simulink model "model6"  (R2022a)
settings: Solver=VariableStepAuto  StartTime=0.0  StopTime=10.0  RelTol=1e-3
values from neighbouring files (symbols this model uses):
  A = [0 0 0 1 0 0; 0 0 0 0 1 0; 0 0 0 0 0 1; 0 6.5 -10 -alpha 0 0; a_51 a_52 a_53 a_54 a_55 a_56; 5 -3.6 0 0 0 -gamma]    [ME5401.m]
  B = [0 0; 0 0; 0 0; beta 11.2; b_51 b_52; 40 delta]    [ME5401.m]    (also in unity_place.m = B*q)
  C = [1 0 0 0 0 0; 0 1 0 0 0 0; 0 0 1 0 0 0]    [ME5401.m]    (also in place_pole.m = CC; unity_place.m = W_c)
  K_2 = my_lqr(A,B,Q,R)    [ME5401.m]
settings Model: Creator=jiaya  LastModifiedBy=jiaya
settings ModelReferenceCC: EnableRefExpFcnMdlSchedulingChecks=off
settings RTWCC: Description=Generic Real-Time Target

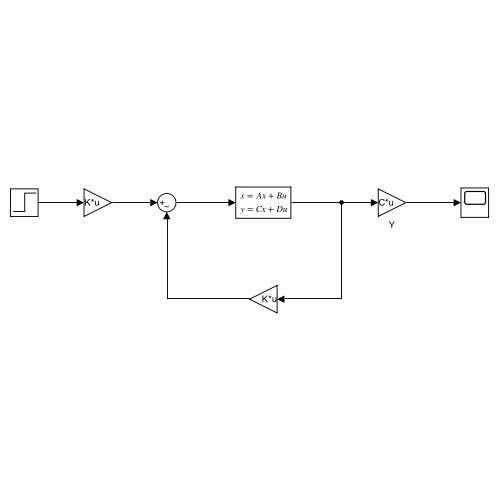
[thumbnail: Simulink's stored preview of the top-level diagram]
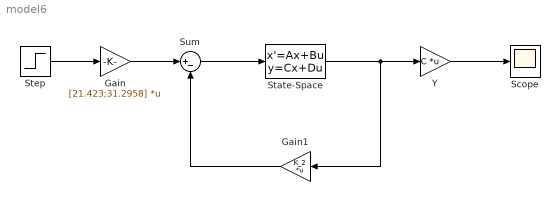
== system model6 ==
  Gain : Gain  Gain=[21.423;31.2958]  Multiplication=Matrix(K*u)
  Gain1 : Gain  Gain=K_2  Multiplication=Matrix(K*u)
  Scope : Scope
  State-Space : StateSpace  A=A  B=B  C=eye(6)  D=zeros(6,2)  InitialCondition=0
  Step : Step  Time=0  SampleTime=0
  Sum : Sum  Inputs=|+-
  Y : Gain  Gain=C  Multiplication=Matrix(K*u)
  wires:
  Sum/1 -> State-Space/1
  Step/1 -> Gain/1
  Gain/1 -> Sum/1
  Gain1/1 -> Sum/2
  State-Space/1 -> Gain1/1, Y/1
  Y/1 -> Scope/1
